simulink model "platoon_closed_v2"  (R2018a)
settings: Solver=VariableStepAuto  StartTime=0.0  StopTime=10  RelTol=1e-3  EnableMultiTasking=on
InitFcn:
  | global mdl;
  | mdl = run_setup_v2;
settings Model: Creator=swsmth  LastModifiedBy=swsmth
settings OptimizationCC: LifeSpan=inf
settings DebuggingCC: SFUnexpectedBacktrackingDiag=warning  SFNoUnconditionalDefaultTransitionDiag=warning  SFExecutionAtInitializationDiag=none
settings CodeAppCC: StateflowObjectComments=on
settings GRTTargetCC: TargetLangStandard=C89/C90 (ANSI)
settings ConfigComp: CovMetricSettings=dw  CovHtmlReporting=on  CovSaveCumulativeToWorkspaceVar=on  CovSaveSingleToWorkspaceVar=on  CovExternalEMLEnable=off

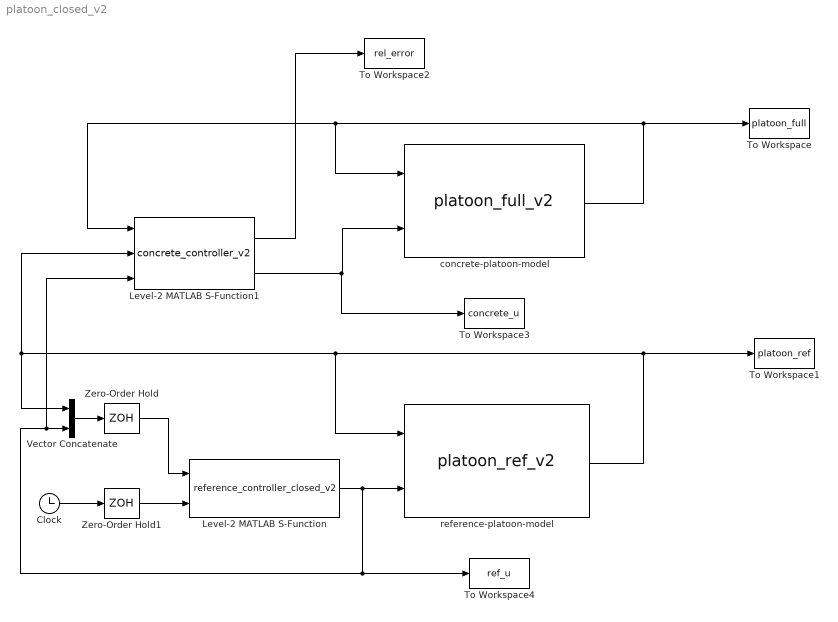
== system platoon_closed_v2 ==
  Clock : Clock
  Level-2 MATLAB S-Function : M-S-Function  FunctionName=reference_controller_closed_v2
  Level-2 MATLAB S-Function1 : M-S-Function  FunctionName=concrete_controller_v2
  To Workspace : ToWorkspace  VariableName=platoon_full  SampleTime=-1
  To Workspace1 : ToWorkspace  VariableName=platoon_ref  SampleTime=-1
  To Workspace2 : ToWorkspace  VariableName=rel_error  SampleTime=-1
  To Workspace3 : ToWorkspace  VariableName=concrete_u  SampleTime=-1
  To Workspace4 : ToWorkspace  VariableName=ref_u  SampleTime=-1
  Vector Concatenate : Concatenate
  Zero-Order Hold : ZeroOrderHold  SampleTime=.1
  Zero-Order Hold1 : ZeroOrderHold  SampleTime=.1
  concrete-platoon-model : M-S-Function  FunctionName=platoon_full_v2
  reference-platoon-model : M-S-Function  FunctionName=platoon_ref_v2
  wires:
  concrete-platoon-model/1 -> Level-2 MATLAB S-Function1/1, concrete-platoon-model/1, To Workspace/1
  reference-platoon-model/1 -> To Workspace1/1, reference-platoon-model/1, Level-2 MATLAB S-Function1/2, Vector Concatenate/1
  Zero-Order Hold/1 -> Level-2 MATLAB S-Function/1
  Level-2 MATLAB S-Function1/1 -> To Workspace2/1
  Level-2 MATLAB S-Function1/2 -> To Workspace3/1, concrete-platoon-model/2
  Level-2 MATLAB S-Function/1 -> Level-2 MATLAB S-Function1/3, Vector Concatenate/2, To Workspace4/1, reference-platoon-model/2
  Vector Concatenate/1 -> Zero-Order Hold/1
  Clock/1 -> Zero-Order Hold1/1
  Zero-Order Hold1/1 -> Level-2 MATLAB S-Function/2
